simulink model "demo_filters_low_and_high_input_chirp"  (Simulink 7.8)
settings: Solver=ode45  StartTime=0.0  StopTime=10.0  RelTol=1e-3
libraries: simulink x1
settings Model: Creator=Ramanathan  LastModifiedBy=Ramanathan

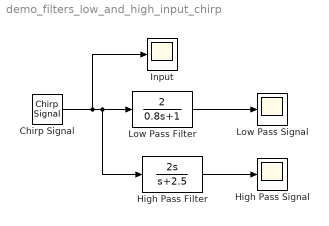
== system demo_filters_low_and_high_input_chirp ==
  Chirp Signal : simulink/Sources/Chirp Signal  f1=0.1  T=100  f2=10
  High Pass Filter : TransferFcn  Numerator=[2 0]  Denominator=[1 2.5]
  High Pass Signal : Scope
      settings: SaveName=ScopeData2
  Input : Scope
  Low Pass Filter : TransferFcn  Numerator=[2]  Denominator=[0.8 1]
  Low Pass Signal : Scope
  wires:
  Low Pass Filter/1 -> Low Pass Signal/1
  Chirp Signal/1 -> Input/1, Low Pass Filter/1, High Pass Filter/1
  High Pass Filter/1 -> High Pass Signal/1
